simulink model "U3"  (R2021a)
settings: Solver=VariableStepAuto  StartTime=0.0  StopTime=20  RelTol=1e-3
libraries: cstblocks x1
settings Model: Creator=wilso  LastModifiedBy=wilso

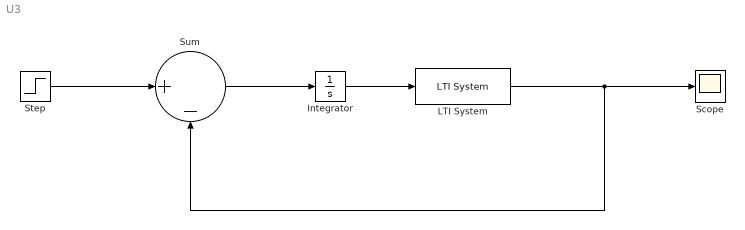
== system U3 ==
  Integrator : Integrator
  LTI System : cstblocks/LTI System  sys=G2  IC=[]
  Scope : Scope
  Step : Step  SampleTime=0
  Sum : Sum  Inputs=|+-
  wires:
  Sum/1 -> Integrator/1
  Integrator/1 -> LTI System/1
  LTI System/1 -> Sum/2, Scope/1
  Step/1 -> Sum/1
